simulink model "A_tenue_pente_filtre_bdg"  (R2019b)
settings: Solver=VariableStepAuto  StartTime=0.0  StopTime=tsim  RelTol=1e-3
undefined symbols (not defined in the file): A_AM, B_AM, C_AM, D_AM, den_BdG, gamma_c, K_gamma, Kn_BdG, Kq, SW_BdG, SW_filtre, tau_filtre_q
settings Model: Creator=Alexa  LastModifiedBy=natha
settings DebuggingCC: SFMachineParentedDataDiag=error

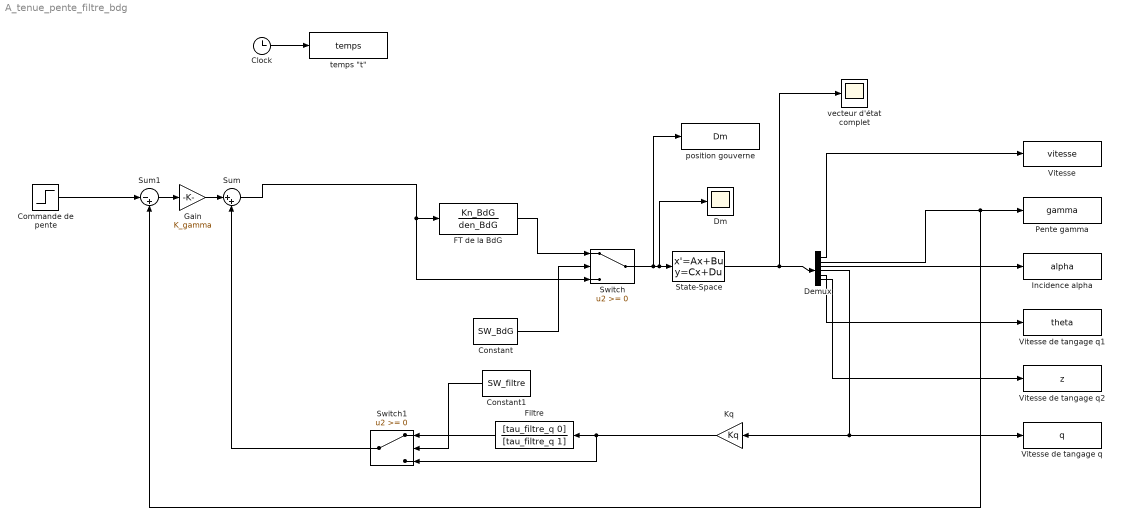
== system A_tenue_pente_filtre_bdg ==
  Clock : Clock
  Commande de pente : Step  Before=gamma_c  After=gamma_c  SampleTime=0
  Constant : Constant  Value=SW_BdG
  Constant1 : Constant  Value=SW_filtre
  Demux : Demux  Outputs=6
  Dm : Scope
  FT de la BdG : TransferFcn  Numerator=Kn_BdG  Denominator=den_BdG
  Filtre : TransferFcn  Numerator=[tau_filtre_q 0]  Denominator=[tau_filtre_q 1]
  Gain : Gain  Gain=K_gamma
  Incidence alpha : ToWorkspace  VariableName=alpha  SampleTime=-1
  Kq : Gain  Gain=Kq
  Pente gamma : ToWorkspace  VariableName=gamma  SampleTime=-1
  State-Space : StateSpace  A=A_AM  B=B_AM  C=C_AM  D=D_AM  InitialCondition=0
  Sum : Sum  Inputs=|++
  Sum1 : Sum  Inputs=|-+
  Switch : Switch
  Switch1 : Switch
  Vitesse : ToWorkspace  VariableName=vitesse  SampleTime=-1
  Vitesse de tangage q : ToWorkspace  VariableName=q  SampleTime=-1
  Vitesse de tangage q1 : ToWorkspace  VariableName=theta  SampleTime=-1
  Vitesse de tangage q2 : ToWorkspace  VariableName=z  SampleTime=-1
  position gouverne : ToWorkspace  VariableName=Dm  SampleTime=-1
  "temps \"t\"" : ToWorkspace  VariableName=temps  SampleTime=-1
  "vecteur d'état complet " : Scope
  wires:
  Switch/1 -> position gouverne/1, Dm/1, State-Space/1
  FT de la BdG/1 -> Switch/1
  State-Space/1 -> Demux/1, "vecteur d'état complet "/1
  Constant/1 -> Switch/2
  Clock/1 -> "temps \"t\""/1
  Switch1/1 -> Sum/2
  Constant1/1 -> Switch1/2
  Filtre/1 -> Switch1/1
  Kq/1 -> Switch1/3, Filtre/1
  Demux/1 -> Vitesse/1
  Demux/2 -> Pente gamma/1, Sum1/2
  Demux/3 -> Incidence alpha/1
  Demux/4 -> Kq/1, Vitesse de tangage q/1
  Sum/1 -> Switch/3, FT de la BdG/1
  Commande de pente/1 -> Sum1/1
  Sum1/1 -> Gain/1
  Gain/1 -> Sum/1
  Demux/5 -> Vitesse de tangage q1/1
  Demux/6 -> Vitesse de tangage q2/1
